simulink model "C2F_K2C_V2K"  (R2020b)
settings: Solver=VariableStepAuto  StartTime=0.0  StopTime=100  RelTol=1e-3
libraries: simulink x1
settings Model: Creator=Training  LastModifiedBy=Training

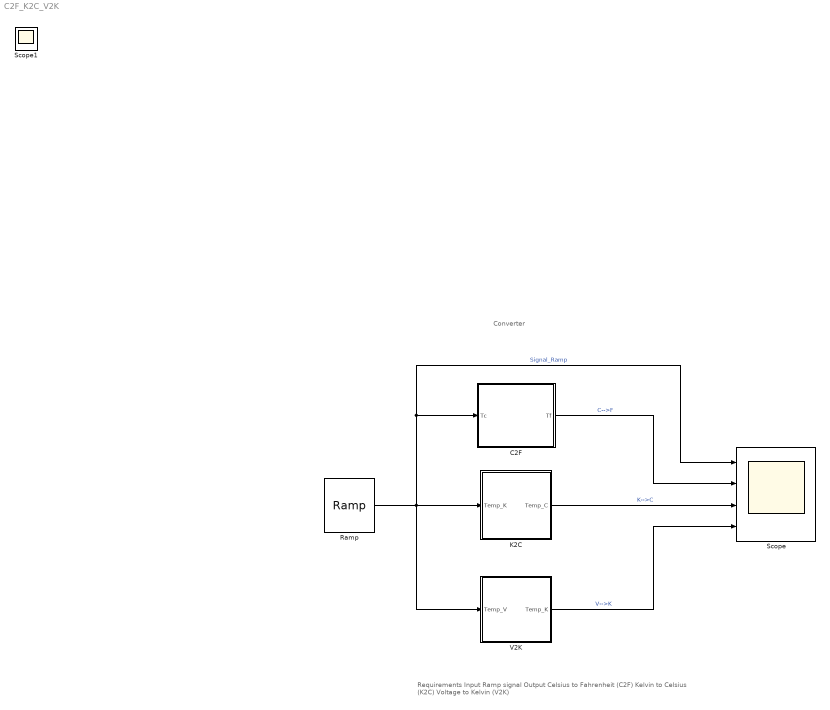
== system C2F_K2C_V2K ==
  note: Requirements
      | Input
      | Ramp signal
      | Output
      | Celsius to Fahrenheit (C2F)
      | Kelvin to Celsius (K2C)
      | Voltage to Kelvin (V2K)
  note: Converter
  C2F : Subsystem
      mask Display: image('C2F.jpg');
  K2C : Subsystem
      mask Display: image('K2C.JPG');
  Ramp : simulink/Sources/Ramp  slope=1  start=0  InitialOutput=-50
  Scope : Scope  NumInputPorts=4
  V2K : Subsystem
      mask Display: image('V2K.PNG');
  Scope1 : Scope
  wires:
  Ramp/1 -> V2K/1(Temp_V), Scope/1, C2F/1(Tc), K2C/1(Temp_K)  "Signal_Ramp"
  C2F/1(Tf) -> Scope/2  "C-->F"
  K2C/1(Temp_C) -> Scope/3  "K-->C"
  V2K/1(Temp_K) -> Scope/4  "V-->K"

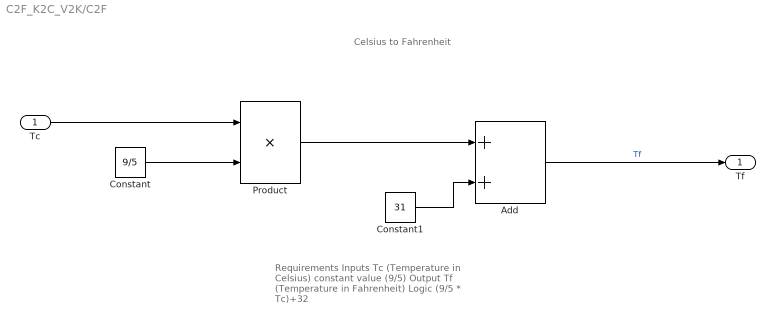
== system C2F_K2C_V2K/C2F ==
  note: Requirements
      | Inputs
      | Tc (Temperature in Celsius)
      | constant value (9/5)
      | Output
      | Tf (Temperature in Fahrenheit)
      | Logic
      | (9/5 * Tc)+32
  note: Celsius to Fahrenheit
  Tc : Inport
  Add : Sum
  Constant : Constant  Value=9/5
  Constant1 : Constant  Value=31
  Product : Product
  Tf : Outport
  wires:
  Constant/1 -> Product/2
  Product/1 -> Add/1
  Tc/1 -> Product/1
  Constant1/1 -> Add/2
  Add/1 -> Tf/1  "Tf"

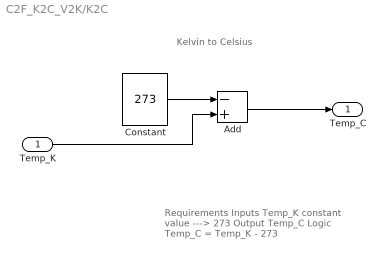
== system C2F_K2C_V2K/K2C ==
  note: Kelvin to Celsius
  note: Requirements
      | Inputs
      | Temp_K
      | constant value ---> 273
      | Output
      | Temp_C
      | Logic
      | Temp_C = Temp_K - 273
  Temp_K : Inport
  Add : Sum  Inputs=-+
  Constant : Constant  Value=273
  Temp_C : Outport
  wires:
  Constant/1 -> Add/1
  Add/1 -> Temp_C/1
  Temp_K/1 -> Add/2

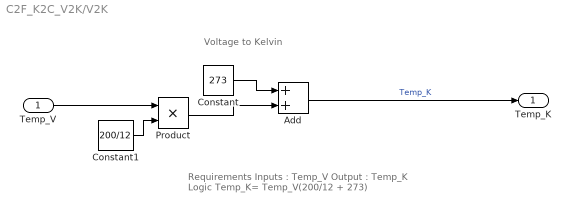
== system C2F_K2C_V2K/V2K ==
  note: Requirements
      | Inputs : Temp_V
      | Output : Temp_K
      | Logic
      | Temp_K= Temp_V(200/12 + 273)
  note: Voltage to Kelvin
  Temp_V : Inport
  Add : Sum
  Constant : Constant  Value=273
  Constant1 : Constant  Value=200/12
  Product : Product
  Temp_K : Outport
  wires:
  Constant/1 -> Add/1
  Add/1 -> Temp_K/1  "Temp_K"
  Constant1/1 -> Product/2
  Product/1 -> Add/2
  Temp_V/1 -> Product/1
